simulink model "PF_IE_1705"  (R2018b)
settings: Solver=FixedStepAuto  StartTime=0.0  StopTime=tfinal  FixedStep=1e-3  RelTol=1e-3
libraries: simulink x2, simulink_extras x2
settings Model: Creator=César  LastModifiedBy=César

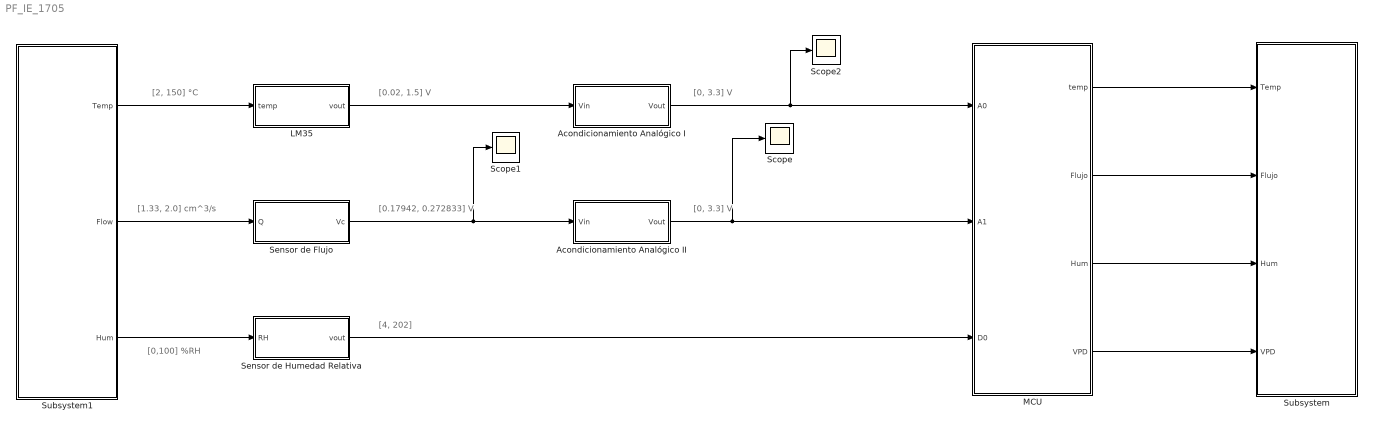
== system PF_IE_1705 ==
  note: [0, 3.3] V
  note: [0.02, 1.5] V
  note: [2, 150] °C
  note: [1.33, 2.0] cm^3/s
  note: [0.17942, 0.272833] V
  note: [0, 3.3] V
  note: [0,100] %RH
  note: [4, 202]
  Acondicionamiento Analógico I : Subsystem  Tag=LM35  Description=Temperature Sensor
  Acondicionamiento Analógico II : Subsystem  Tag=LM35  Description=Temperature Sensor
  LM35 : Subsystem  Tag=LM35  Description=Temperature Sensor
  MCU : Subsystem  Tag=LM35  Description=Temperature Sensor
  Scope : Scope
  Scope1 : Scope
  Scope2 : Scope
  Sensor de Flujo : Subsystem  Tag=LM35  Description=Temperature Sensor
  Sensor de Humedad Relativa : Subsystem  Tag=LM35  Description=Temperature Sensor
  Subsystem : Subsystem
  Subsystem1 : Subsystem
  wires:
  Subsystem1/1(Temp) -> LM35/1("temp ")
  Acondicionamiento Analógico I/1("Vout ") -> Scope2/1, MCU/1("A0 ")
  Sensor de Humedad Relativa/1("vout ") -> MCU/3("D0 ")
  Subsystem1/3(Hum) -> Sensor de Humedad Relativa/1("RH ")
  Subsystem1/2(Flow) -> Sensor de Flujo/1("Q ")
  Acondicionamiento Analógico II/1("Vout ") -> Scope/1, MCU/2("A1 ")
  Sensor de Flujo/1("Vc ") -> Scope1/1, Acondicionamiento Analógico II/1("Vin ")
  LM35/1("vout ") -> Acondicionamiento Analógico I/1("Vin ")
  MCU/1("temp ") -> Subsystem/1(Temp)
  MCU/2(Flujo) -> Subsystem/2(Flujo)
  MCU/3("Hum ") -> Subsystem/3(Hum)
  MCU/4(VPD) -> Subsystem/4(VPD)

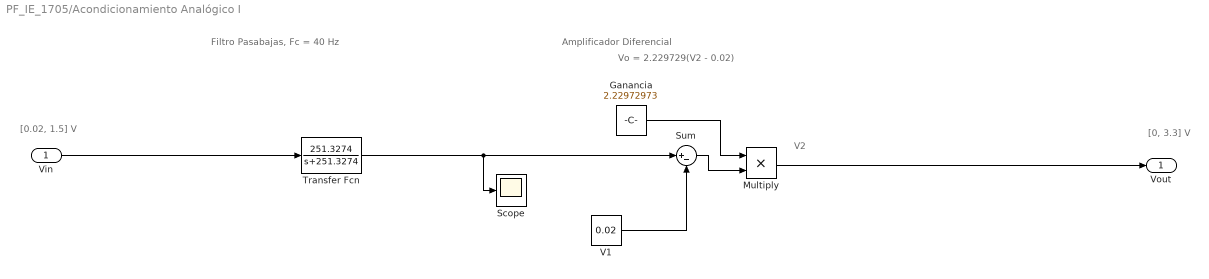
== system PF_IE_1705/Acondicionamiento Analógico I ==
  note: Vo = 2.229729(V2 - 0.02)
  note: V2
  note: [0, 3.3] V
  note: Amplificador Diferencial
  note: [0.02, 1.5] V
  note: Filtro Pasabajas, Fc = 40 Hz
  "Vin " : Inport
  "Ganancia " : Constant  Value=2.22972973
  Multiply : Product
  Scope : Scope
  Sum : Sum  Inputs=|+-
  Transfer Fcn : TransferFcn  Numerator=[251.3274]  Denominator=[1 251.3274]
  V1 : Constant  Value=0.02
  "Vout " : Outport
  wires:
  V1/1 -> Sum/2
  "Ganancia "/1 -> Multiply/1
  Sum/1 -> Multiply/2
  "Vin "/1 -> Transfer Fcn/1
  Transfer Fcn/1 -> Scope/1, Sum/1
  Multiply/1 -> "Vout "/1

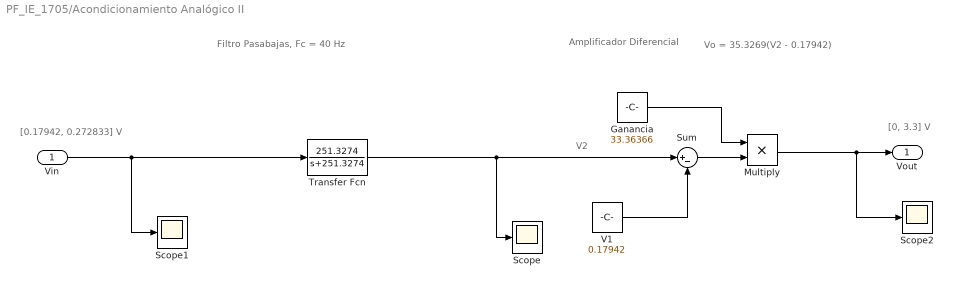
== system PF_IE_1705/Acondicionamiento Analógico II ==
  note: Vo = 35.3269(V2 - 0.17942)
  note: V2
  note: [0, 3.3] V
  note: Amplificador Diferencial
  note: [0.17942, 0.272833] V
  note: Filtro Pasabajas, Fc = 40 Hz
  "Vin " : Inport
  "Ganancia " : Constant  Value=33.36366
  Multiply : Product
  Scope : Scope
  Scope1 : Scope
  Scope2 : Scope
  Sum : Sum  Inputs=|+-
  Transfer Fcn : TransferFcn  Numerator=[251.3274]  Denominator=[1 251.3274]
  V1 : Constant  Value=0.17942
  "Vout " : Outport
  wires:
  Multiply/1 -> Scope2/1, "Vout "/1
  V1/1 -> Sum/2
  "Ganancia "/1 -> Multiply/1
  Sum/1 -> Multiply/2
  "Vin "/1 -> Scope1/1, Transfer Fcn/1
  Transfer Fcn/1 -> Scope/1, Sum/1

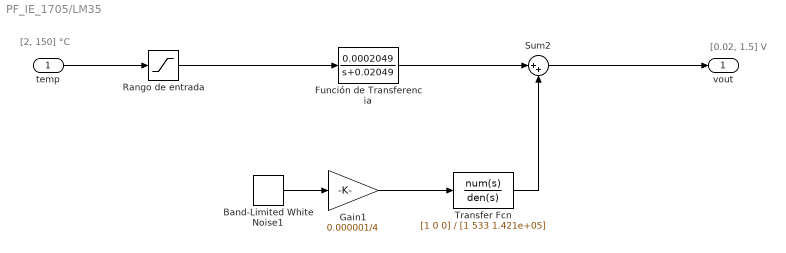
== system PF_IE_1705/LM35 ==
  note: [0.02, 1.5] V
  note: [2, 150] °C
  "temp " : Inport
  Band-Limited White Noise1 : simulink/Sources/Band-Limited White Noise  Cov=[1]  Ts=1e-3  seed=[23341]
  Función de Transferencia : TransferFcn  Numerator=[0.0002049]  Denominator=[1 0.02049]
  Gain1 : Gain  Gain=0.000001/4
  Rango de entrada : Saturate  UpperLimit=150  LowerLimit=2
  Sum2 : Sum  Inputs=|++
  Transfer Fcn : TransferFcn  Numerator=[1 0 0]  Denominator=[1 533 1.421e+05]
  "vout " : Outport
  wires:
  Rango de entrada/1 -> Función de Transferencia/1
  Función de Transferencia/1 -> Sum2/1
  "temp "/1 -> Rango de entrada/1
  Sum2/1 -> "vout "/1
  Band-Limited White Noise1/1 -> Gain1/1
  Transfer Fcn/1 -> Sum2/2
  Gain1/1 -> Transfer Fcn/1

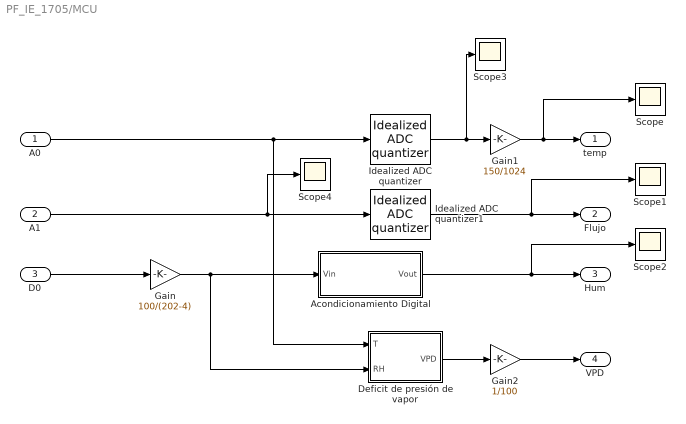
== system PF_IE_1705/MCU ==
  "A0 " : Inport
  "A1 " : Inport  Port=2
  "D0 " : Inport  Port=3
  "Acondicionamiento Digital " : Subsystem  Tag=LM35  Description=Temperature Sensor
  Deficit de presión de vapor : MATLAB Function  TreatAsAtomicUnit=on
  Gain : Gain  Gain=100/(202-4)
  Gain1 : Gain  Gain=150/1024
  Gain2 : Gain  Gain=1/100
  Idealized ADC quantizer : simulink_extras/Additional Discrete/Idealized ADC quantizer  NumberOfConverterBits=10  Vmin=0  Vmax=3.3  OutputDataType=int16  OutputNegativeValues=off
      settings: SourceProductName=Simulink
  Idealized ADC quantizer1 : simulink_extras/Additional Discrete/Idealized ADC quantizer  NumberOfConverterBits=10  Vmin=0  Vmax=3.3  OutputDataType=int16  OutputNegativeValues=off
      settings: SourceProductName=Simulink
  Scope{,1..4} (5 alike) : Scope
  "temp " : Outport
  Flujo : Outport  Port=2
  "Hum " : Outport  Port=3
  VPD : Outport  Port=4
  wires:
  "A0 "/1 -> Idealized ADC quantizer/1, Deficit de presión de vapor/1(T)
  "Acondicionamiento Digital "/1("Vout ") -> Scope2/1, "Hum "/1
  "A1 "/1 -> Scope4/1, Idealized ADC quantizer1/1
  "D0 "/1 -> Gain/1
  Gain/1 -> Deficit de presión de vapor/2(RH), "Acondicionamiento Digital "/1("Vin ")
  Deficit de presión de vapor/1(VPD) -> Gain2/1
  Gain2/1 -> VPD/1
  Idealized ADC quantizer1/1 -> Scope1/1, Flujo/1
  Idealized ADC quantizer/1 -> Scope3/1, Gain1/1
  Gain1/1 -> Scope/1, "temp "/1

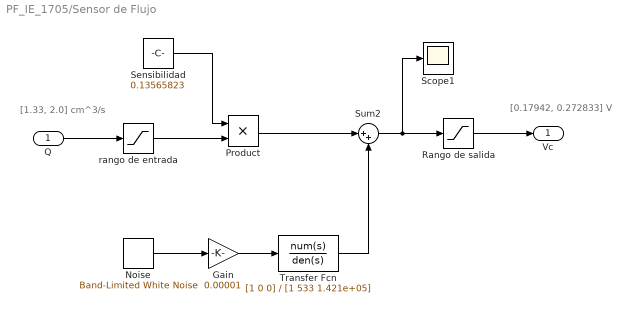
== system PF_IE_1705/Sensor de Flujo ==
  note: [1.33, 2.0] cm^3/s
  note: [0.17942, 0.272833] V
  "Q " : Inport
  Gain : Gain  Gain=0.00001
  Noise : simulink/Sources/Band-Limited White Noise  Cov=[0.01]  Ts=1e-3  seed=[23341]
  Product : Product
  Rango de salida : Saturate  UpperLimit=0.28  LowerLimit=0.16
  Scope1 : Scope
  Sensibilidad : Constant  Value=0.13565823
  Sum2 : Sum  Inputs=|++
  Transfer Fcn : TransferFcn  Numerator=[1 0 0]  Denominator=[1 533 1.421e+05]
  rango de entrada : Saturate  UpperLimit=2.0  LowerLimit=1.32
  "Vc " : Outport
  wires:
  Sensibilidad/1 -> Product/1
  "Q "/1 -> rango de entrada/1
  rango de entrada/1 -> Product/2
  Sum2/1 -> Scope1/1, Rango de salida/1
  Product/1 -> Sum2/1
  Noise/1 -> Gain/1
  Rango de salida/1 -> "Vc "/1
  Gain/1 -> Transfer Fcn/1
  Transfer Fcn/1 -> Sum2/2

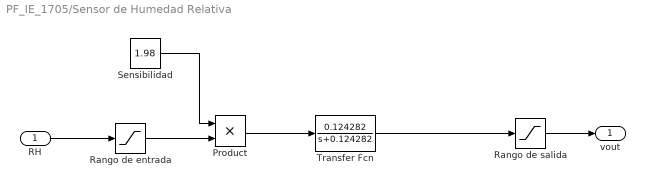
== system PF_IE_1705/Sensor de Humedad Relativa ==
  "RH " : Inport
  Product : Product
  Rango de entrada : Saturate  UpperLimit=100  LowerLimit=0
  Rango de salida : Saturate  UpperLimit=255  LowerLimit=0
  Sensibilidad : Constant  Value=1.98
  Transfer Fcn : TransferFcn  Numerator=[0.124282]  Denominator=[1 0.124282]
  "vout " : Outport
  wires:
  Product/1 -> Transfer Fcn/1
  Sensibilidad/1 -> Product/1
  "RH "/1 -> Rango de entrada/1
  Rango de entrada/1 -> Product/2
  Rango de salida/1 -> "vout "/1
  Transfer Fcn/1 -> Rango de salida/1

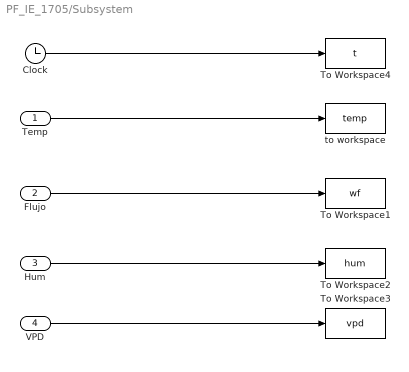
== system PF_IE_1705/Subsystem ==
  Temp : Inport
  Flujo : Inport  Port=2
  Hum : Inport  Port=3
  VPD : Inport  Port=4
  Clock : Clock
  To Workspace1 : ToWorkspace  VariableName=wf  SampleTime=-1
  To Workspace2 : ToWorkspace  VariableName=hum  SampleTime=-1
  To Workspace3 : ToWorkspace  VariableName=vpd  SampleTime=-1
  To Workspace4 : ToWorkspace  VariableName=t  SampleTime=-1
  to workspace : ToWorkspace  VariableName=temp  SampleTime=-1
  wires:
  Temp/1 -> to workspace/1
  Flujo/1 -> To Workspace1/1
  Hum/1 -> To Workspace2/1
  VPD/1 -> To Workspace3/1
  Clock/1 -> To Workspace4/1

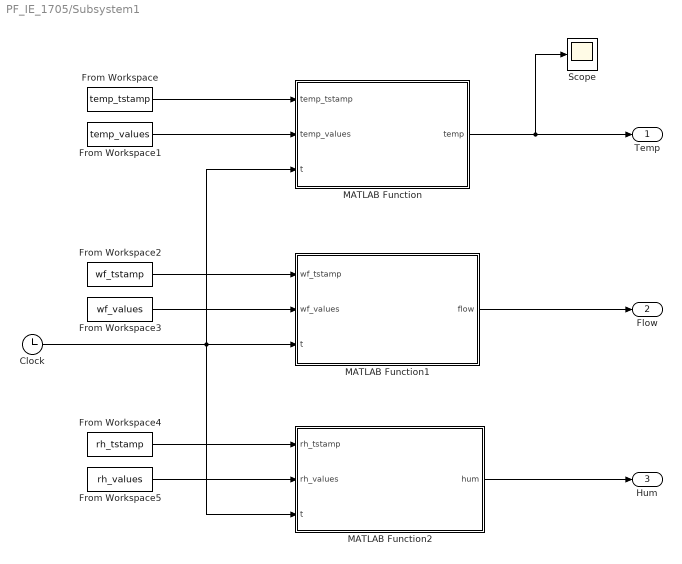
== system PF_IE_1705/Subsystem1 ==
  Clock : Clock
  From Workspace : FromWorkspace  VariableName=temp_tstamp  SampleTime=0
  From Workspace1 : FromWorkspace  VariableName=temp_values  SampleTime=0
  From Workspace2 : FromWorkspace  VariableName=wf_tstamp  SampleTime=0
  From Workspace3 : FromWorkspace  VariableName=wf_values  SampleTime=0
  From Workspace4 : FromWorkspace  VariableName=rh_tstamp  SampleTime=0
  From Workspace5 : FromWorkspace  VariableName=rh_values  SampleTime=0
  MATLAB Function : MATLAB Function  TreatAsAtomicUnit=on
  MATLAB Function1 : MATLAB Function  TreatAsAtomicUnit=on
  MATLAB Function2 : MATLAB Function  TreatAsAtomicUnit=on
  Scope : Scope
  Temp : Outport
  Flow : Outport  Port=2
  Hum : Outport  Port=3
  wires:
  MATLAB Function1/1(flow) -> Flow/1
  MATLAB Function2/1(hum) -> Hum/1
  Clock/1 -> MATLAB Function/3(t), MATLAB Function2/3(t), MATLAB Function1/3(t)
  MATLAB Function/1(temp) -> Scope/1, Temp/1
  From Workspace/1 -> MATLAB Function/1(temp_tstamp)
  From Workspace1/1 -> MATLAB Function/2(temp_values)
  From Workspace2/1 -> MATLAB Function1/1(wf_tstamp)
  From Workspace3/1 -> MATLAB Function1/2(wf_values)
  From Workspace4/1 -> MATLAB Function2/1(rh_tstamp)
  From Workspace5/1 -> MATLAB Function2/2(rh_values)

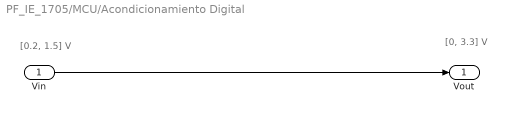
== system PF_IE_1705/MCU/Acondicionamiento Digital  ==
  note: [0, 3.3] V
  note: [0.2, 1.5] V
  "Vin " : Inport
  "Vout " : Outport
  wires:
  "Vin "/1 -> "Vout "/1

== matlab function PF_IE_1705/Subsystem1/MATLAB Function ==
  data: temp_tstamp input; temp_values input; t input; temp output
function temp = fcn(temp_tstamp, temp_values, t)
if(t/60 < temp_tstamp(1))
    temp = temp_values(1);
elseif(t/60 < temp_tstamp(2))
    temp = temp_values(2);
elseif(t/60 < temp_tstamp(3))
    temp = temp_values(3);
elseif(t/60 > temp_tstamp(4))
    temp = temp_values(4);
else
    temp = temp_values(4);
end

== matlab function PF_IE_1705/MCU/Deficit de presión de vapor ==
  data: T input; VPD output; RH input
function VPD = fcn(T,RH)

VPD = exp(6.41+(0.0727*T)-(3e-4*(T^2))+(1.18e-6*(T^3))-(3.86e-9*(T^4)))*(1-(RH/100));

== matlab function PF_IE_1705/Subsystem1/MATLAB Function1 ==
  data: wf_tstamp input; wf_values input; t input; flow output
function flow = fcn(wf_tstamp, wf_values, t)

if(t/60 < wf_tstamp(1))
    flow = wf_values(1);
elseif(t/60 < wf_tstamp(2))
    flow = wf_values(2);
elseif(t/60 < wf_tstamp(3))
    flow = wf_values(3);
elseif(t/60 > wf_tstamp(4))
    flow = wf_values(4);
else
    flow = wf_values(4);
end

== matlab function PF_IE_1705/Subsystem1/MATLAB Function2 ==
  data: rh_tstamp input; rh_values input; t input; hum output
function hum = fcn(rh_tstamp, rh_values, t)

if(t/60 < rh_tstamp(1))
    hum = rh_values(1);
elseif(t/60 < rh_tstamp(2))
    hum = rh_values(2);
elseif(t/60 < rh_tstamp(3))
    hum = rh_values(3);
elseif(t/60 > rh_tstamp(4))
    hum = rh_values(4);
else
    hum = rh_values(4);
end
